simulink model "sraam2023b"  (R2023b)
settings: Solver=ode4  StartTime=0.0  StopTime=25  FixedStep=0.001  RelTol=1e-3
values from neighbouring files (symbols this model uses):
  AEXIT = 0.0125    [SRAAM6_params.m]
  ALIMIT = 50.0    (= 50)    [SRAAM6_params.m]
  ALP_LIMX = 46.0    (= 46)    [SRAAM6_params.m]
  BIASAL = 0.0    (= 0)    [SRAAM6_params.m]
  DDLIMX = 600.0    (= 600)    [SRAAM6_params.m]
  DLIMX = 28.0    (= 28)    [SRAAM6_params.m]
  DPLIMX = 28.0    (= 28)    [SRAAM6_params.m]
  DQLIMX = 28.0    (= 28)    [SRAAM6_params.m]
  DRLIMX = 28.0    (= 28)    [SRAAM6_params.m]
  DT = 0.001    [SRAAM6_params.m]
  EBIASA = zeros(3,1)    [SRAAM6_params.m]
  EBIASG = zeros(3,1)    [SRAAM6_params.m]
  EMISA = zeros(3,1)    [SRAAM6_params.m]
  EMISG = zeros(3,1)    [SRAAM6_params.m]
  ESCALA = zeros(3,1)    [SRAAM6_params.m]
  ESCALG = zeros(3,1)    [SRAAM6_params.m]
  EUNBG = zeros(3,1)    [SRAAM6_params.m]
  FACT_WRCL = 0.0    (= 0)    [SRAAM6_params.m]
  GNAV = 4.0    (= 4)    [SRAAM6_params.m]
  INS_NOISE_PWR_A = 0.0    (= 0)    [SRAAM6_params.m]
  INS_NOISE_PWR_G = 0.0    (= 0)    [SRAAM6_params.m]
  K_ALPHA = 10.0    (= 10)    [SRAAM6_params.m]
  K_BETA = 10.0    (= 10)    [SRAAM6_params.m]
  MINS = 0    [SRAAM6_params.m]
  prop_cg_t = prop_cg_vs_time_t(:)    [SRAAM6_params.m]
  prop_cg_v = prop_cg_vs_time_v(:)    [SRAAM6_params.m]
  prop_mass_t = prop_mass_vs_time_t(:)    [SRAAM6_params.m]
  prop_mass_v = prop_mass_vs_time_v(:)    [SRAAM6_params.m]
  prop_moipitch_t = prop_moipitch_vs_time_t(:)    [SRAAM6_params.m]
  prop_moipitch_v = prop_moipitch_vs_time_v(:)    [SRAAM6_params.m]
  prop_moiroll_t = prop_moiroll_vs_time_t(:)    [SRAAM6_params.m]
  prop_moiroll_v = prop_moiroll_vs_time_v(:)    [SRAAM6_params.m]
  prop_thrust_t = prop_thrust_vs_time_t(:)    [SRAAM6_params.m]
  prop_thrust_v = prop_thrust_vs_time_v(:)    [SRAAM6_params.m]
  REFA = 0.01824    [SRAAM6_params.m]
  REFL = 0.1524    [SRAAM6_params.m]
  SCENARIO = 12    [SRAAM6_params.m]
  TGET_POS_IC = TGET_POS(SCENARIO, :)'    [SRAAM6_params.m]
  TGET_VEL_IC = TGET_VEL(SCENARIO, :)'    [SRAAM6_params.m]
  WBLIMX = 30.0    (= 30)    [SRAAM6_params.m]
  WN_NDI_Q = 50.0    (= 50)    [SRAAM6_params.m]
  WN_NDI_R = 50.0    (= 50)    [SRAAM6_params.m]
  WNACT = 251.0    (= 251)    [SRAAM6_params.m]
  X_IC = [SBEL_INIT; VBEB_IC; Q_IC; OMEGA_IC]    [SRAAM6_params.m]
  XCG_REF = 1.2994    [SRAAM6_params.m]
  ZETACT = 0.7    [SRAAM6_params.m]
  ZRCL = 0.9    [SRAAM6_params.m]
undefined symbols (not defined in the file or in its folder): alpha_bp, beta_bp, ca0_vs_mach, ca0b_vs_mach, caa_vs_mach_alpha_beta, cad_vs_mach, cll0_vs_mach_alpha_beta, clldp_vs_mach_alpha_beta, cllp_vs_mach, clm0_vs_mach_alpha_beta, clmdq_vs_mach_alpha_beta, clmq_vs_mach, cln0_vs_mach_alpha_beta, clndr_vs_mach_alpha_beta, clnr_vs_mach, cn0_vs_mach_alpha_beta, cndq_vs_mach_alpha_beta, cy0_vs_mach_alpha_beta, cydr_vs_mach_alpha_beta, mach_bp
libraries: simulink x3
(part 2 of 2)

== matlab function sraam2023b/Control Subsystem/NDI ==
  data: ancomx input; dqcx output; alcomx input; alphax input; betax input; dvbe input; qqx input; rrx input; fspb2 input; fspb3 input; dna input; dma input; dmq input; dmd input; dyb input; dlnb input; dlnr input; dlnd input; drcx output; ALIMIT parameter; ALP_LIMX parameter; WBLIMX parameter; DQLIMX parameter; DRLIMX parameter; WN_NDI_Q parameter; WN_NDI_R parameter; K_ALPHA parameter; K_BETA parameter
function [dqcx, drcx] = control_ndi( ...
    ancomx, alcomx, ...
    alphax, betax, dvbe, ...
    qqx, rrx, ...
    fspb2, fspb3, ...
    dna, dma, dmq, dmd, dyb, dlnb, dlnr, dlnd, ALIMIT, ALP_LIMX, WBLIMX, DQLIMX, DRLIMX, WN_NDI_Q, WN_NDI_R, K_ALPHA, K_BETA)
% qqx, rrx: deg/s — kinBus'tan direkt
%CONTROL_NDI  Nonlinear Dynamic Inversion — yunuslama + yalpalama.
% Kaynak: missile/control.py — control_ndi()
% Roll ayrı subsystem'de (control_roll.m).
%#codegen

AGRAV  = 9.80665;
DEG    = 180.0 / pi;
RAD    = pi / 180.0;
SMALL  = 1e-7;

alimit   = ALIMIT;
alplimx  = ALP_LIMX;
wblimx   = WBLIMX;
dqlimx   = DQLIMX;
drlimx   = DRLIMX;
wn_ndi_q = WN_NDI_Q;
wn_ndi_r = WN_NDI_R;
k_alpha  = K_ALPHA;
k_beta   = K_BETA;

% ── Yapısal ivme sınırlayıcı ─────────────────────────────────────────────────
aa = sqrt(ancomx^2 + alcomx^2);
if aa > alimit;  aa = alimit;  end
if abs(ancomx) < SMALL && abs(alcomx) < SMALL
    phi_c = 0.0;
else
    phi_c = atan2(ancomx, alcomx);
end
alcomx_l = aa * cos(phi_c);
ancomx_l = aa * sin(phi_c);

% ── ADIM 1: Kuvvet inversiyonu ────────────────────────────────────────────────
dna_s = dna; if abs(dna_s) < SMALL; dna_s = SMALL; end
dyb_s = dyb; if abs(dyb_s) < SMALL; dyb_s = SMALL; end

alpha_cmd = AGRAV * ancomx_l / dna_s;
beta_cmd  = AGRAV * alcomx_l / dyb_s;

alp_lim   = alplimx * RAD;
alpha_cmd = max(min(alpha_cmd, alp_lim), -alp_lim);
beta_cmd  = max(min(beta_cmd,  alp_lim), -alp_lim);

% ── ADIM 2: Kinematik inversiyon ──────────────────────────────────────────────
alpha   = alphax * RAD;
beta    = betax  * RAD;
qq      = qqx * RAD;    % deg/s → rad/s
rr      = rrx * RAD;
V_s     = max(dvbe, 30.0);
an_meas = -fspb3 / AGRAV;
al_meas =  fspb2 / AGRAV;

q_cmd = k_alpha * (alpha_cmd - alpha) + AGRAV * an_meas / V_s;
r_cmd = k_beta  * (beta - beta_cmd)   + AGRAV * al_meas / V_s;

rate_lim = wblimx * RAD;
q_cmd = max(min(q_cmd, rate_lim), -rate_lim);
r_cmd = max(min(r_cmd, rate_lim), -rate_lim);

% ── ADIM 3: Moment inversiyonu ────────────────────────────────────────────────
q_dot_des   = wn_ndi_q * (q_cmd - qq);
r_dot_des   = wn_ndi_r * (r_cmd - rr);
q_dot_model = dma * alpha + dmq * qq;
r_dot_model = dlnb * beta + dlnr * rr;

dmd_s  = dmd;  if abs(dmd_s)  < SMALL; dmd_s  = SMALL; end
dlnd_s = dlnd; if abs(dlnd_s) < SMALL; dlnd_s = SMALL; end

dqc  = (q_dot_des - q_dot_model) / dmd_s;
drc  = (r_dot_des - r_dot_model) / dlnd_s;

dqcx = max(min(dqc * DEG, dqlimx), -dqlimx);
drcx = max(min(drc * DEG, drlimx), -drlimx);
end

== matlab function sraam2023b/Target/Target ==
  data: t input; acc output; pos input; vel input; scenario input
function acc = target_accel(t, pos, vel, scenario)
%TARGET_ACCEL  Hedef ivme vektörü — 10 senaryo.
% Kaynak: missile/target.py — Target._accel()
%
% Girişler:
%   t        : simülasyon zamanı - s
%   pos      : hedef konumu NED - m  (kullanılmıyor, ileriki senaryolar için)
%   vel      : hedef hızı NED - m/s
%   scenario : senaryo numarası (1-10)
%
% Çıkış:
%   acc [3x1]: hedef ivmesi NED - m/s²
%#codegen

G = 9.80665;
acc = zeros(3,1);

vn = vel(1);  ve = vel(2);  vd = vel(3);

% ── Yardımcı: saat yönünde dik vektör (yatay düzlemde) ───────────────────────
vm = sqrt(vn^2 + ve^2);
if vm < 1.0
    cw_n = 0.0;  cw_e = 0.0;
else
    cw_n =  ve / vm;
    cw_e = -vn / vm;
end

if scenario == 1
    % S1: Sabit hız, düz uçuş
    acc = zeros(3,1);

elseif scenario == 2
    % S2: t>1.5s'de 5g sağ kırılma (santripetal)
    if t >= 1.5
        acc = 5.0 * G * [cw_n; cw_e; 0.0];
    end

elseif scenario == 3
    % S3: Sinüsoidal manevra (3g yanal + 2g dikey)
    acc = [0.0; 3.0*G*sin(1.2*t); -2.0*G*cos(1.8*t + pi/3)];

elseif scenario == 4
    % S4: t>2s 8g sağ kırılma, t>3.5s 6g yukarı çekme
    if t >= 4.8
        acc = zeros(3,1);
    elseif t >= 3.5
        acc = [0.0; 0.0; -6.0*G];
    elseif t >= 2.0
        acc = 8.0 * G * [cw_n; cw_e; 0.0];
    end

elseif scenario == 5
    % S5: Sabit hız (beaming)
    acc = zeros(3,1);

elseif scenario == 6
    % S6: t>3s 7g sağ kırılma, t>8s düzleşme
    if t >= 8.0
        acc = zeros(3,1);
    elseif t >= 3.0
        acc = 7.0 * G * [cw_n; cw_e; 0.0];
    end

elseif scenario == 7
    % S7: Sabit hız (look-down)
    acc = zeros(3,1);

elseif scenario == 8
    % S8: t>4s ~9g kombine kırılma
    if t >= 4.0
        acc = [0.0; 6.364*G; -6.364*G];
    end

elseif scenario == 9
    % S9: Afterburner tırmanma (~3g)
    vtot = norm(vel);
    if vtot > 1.0
        vhat = vel / vtot;
        a_drag = -0.7 * G * vhat;
        up = [0.0; 0.0; -1.0];
        perp = up - dot(up, vhat) * vhat;
        pm = norm(perp);
        if pm > 1e-6
            a_lift = 3.0 * G * perp / pm;
        else
            a_lift = zeros(3,1);
        end
        acc = a_drag + a_lift;
    end

elseif scenario == 10
    % S10: 4g koordineli dönüş
    vm2 = sqrt(vn^2 + ve^2);
    if vm2 > 0.1
        ax = -vel(2) / vm2 * 4.0 * G;
        ay =  vel(1) / vm2 * 4.0 * G;
        acc = [ax; ay; 0.0];
    end

elseif scenario == 11
    % S11: 12km + t>7s geç 6g sağ kırılma
    if t >= 7.0
        acc = 6.0 * G * [cw_n; cw_e; 0.0];
    end

elseif scenario == 12
    % S12: 15km + t>5s sinüsoidal jink (3g yanal + 2g dikey)
    if t >= 5.0
        tau = t - 5.0;
        acc = [0.0; 3.0*G*sin(1.0*tau); -2.0*G*cos(1.5*tau)];
    end

elseif scenario == 13
    % S13: Tail-chase + t>4s 7g yukarı + t>6s 7g sağ kırılma
    if t >= 6.0
        acc = 7.0 * G * [cw_n; cw_e; 0.0];
    elseif t >= 4.0
        acc = [0.0; 0.0; -7.0*G];
    end

elseif scenario == 14
    % S14: Uzun beam + t>6s 8g sharp break
    if t >= 6.0
        acc = 8.0 * G * [cw_n; cw_e; 0.0];
    end
end
end

== matlab function sraam2023b/Guidance Subsystem/guidance ==
  data: STEL input; ancomx output; VTEL input; SBELC input; VBELC input; TBL input; alcomx output; dtbc output; tgoc output; GNAV parameter; ALIMIT parameter
function [ancomx, alcomx, dtbc, tgoc] = guidance_pronav( ...
    STEL, VTEL, SBELC, VBELC, TBL, GNAV, ALIMIT)
%GUIDANCE_PRONAV  Orantılı navigasyon güdümü (midcourse pronav).
% Kaynak: missile/guidance.py — _pronav_mid()
%
% Girişler:
%   STEL  [3x1] : hedef konumu NED - m
%   VTEL  [3x1] : hedef hızı NED - m/s
%   SBELC [3x1] : füze konumu (INS tahmini) NED - m
%   VBELC [3x1] : füze hızı (INS tahmini) NED - m/s
%   TBL   [3x3] : gövde-yerel DCM (INS tahmini)
%
% Çıkışlar:
%   ancomx : normal ivme komutu - g
%   alcomx : yanal ivme komutu - g
%   dtbc   : hedefe mesafe - m
%   tgoc   : tahmini uçuş süresi - s
%#codegen

AGRAV = 9.80665;
SMALL = 1e-7;
gnav  = GNAV;     % workspace parametresi
alimit = ALIMIT;  % workspace parametresi

ancomx = 0.0;
alcomx = 0.0;
dtbc   = 0.0;
tgoc   = 0.0;

% ── Hedef-füze görüş vektörü ──────────────────────────────────────────────────
STBLC = STEL - SBELC;
dtbc  = norm(STBLC);

if dtbc < SMALL
    return
end

UTBLC = STBLC / dtbc;

% ── Görüş açısı (diagnostik) ─────────────────────────────────────────────────
% UTBBC = TBL * UTBLC;  (ileride kullanılabilir)

% ── Göreceli hız (hedef - füze) ───────────────────────────────────────────────
VTBLC = VTEL - VBELC;

% ── Kapanma hızı ─────────────────────────────────────────────────────────────
dvtbc = abs(dot(UTBLC, VTBLC));
if dvtbc < SMALL; dvtbc = SMALL; end

% ── Tahmini uçuş süresi ───────────────────────────────────────────────────────
tgoc = dtbc / dvtbc;

% ── Eylemsiz LOS açısal hızı ─────────────────────────────────────────────────
WOELC = cross(UTBLC, VTBLC) / dtbc;

% ── ProNav ivme komutu (gövde ekseni) - g ────────────────────────────────────
ACBX = TBL * cross(WOELC, UTBLC) * gnav * dvtbc / AGRAV;

% ── Yanal ve normal bileşenler ────────────────────────────────────────────────
all_acc =  ACBX(2);
ann_acc = -ACBX(3);

% ── Dairesel sınırlayıcı ─────────────────────────────────────────────────────
aa = sqrt(all_acc^2 + ann_acc^2);
if aa > alimit;  aa = alimit;  end
if abs(ann_acc) < SMALL && abs(all_acc) < SMALL
    phi = 0.0;
else
    phi = atan2(ann_acc, all_acc);
end

alcomx = aa * cos(phi);
ancomx = aa * sin(phi);
end

== matlab function sraam2023b/Hit Condition ==
  data: dtbc input; stop output; t input; HIT_R parameter
function stop = hit_condition(dtbc, t, HIT_R)
%HIT_CONDITION  HIT_R > 0 ise dtbc < HIT_R olduğunda 1 döndürür.
%#codegen

hit_r = HIT_R;   % workspace parametresi (0 = devre dışı)

if hit_r > 0 && dtbc < hit_r && dtbc > 0 && t > 0.1
    stop = 1.0;
else
    stop = 0.0;
end
end

== matlab function sraam2023b/Control Subsystem/NDI-COP ==
  data: ancomx input; dqcx output; alcomx input; alphax input; betax input; dvbe input; qqx input; rrx input; fspb2 input; fspb3 input; dna input; dma input; dmq input; dmd input; dnd input; dyb input; dlnb input; dlnr input; dlnd input; drcx output; ALIMIT parameter; ALP_LIMX parameter; WBLIMX parameter; DQLIMX parameter; DRLIMX parameter; WN_NDI_Q parameter; WN_NDI_R parameter; K_ALPHA parameter; K_BETA parameter
function [dqcx, drcx] = control_ndi_cop( ...
    ancomx, alcomx, ...
    alphax, betax, dvbe, ...
    qqx, rrx, ...
    fspb2, fspb3, ...
    dna, dma, dmq, dmd, dnd, dyb, dlnb, dlnr, dlnd, ALIMIT, ALP_LIMX, WBLIMX, DQLIMX, DRLIMX, WN_NDI_Q, WN_NDI_R, K_ALPHA, K_BETA)
%CONTROL_NDI_COP  NDI autopilot reformulated about the Center of Percussion.
%
% Kaynak: missile/control.py — control_ndi_cop()  (maut=7)
%
% Standart NDI'dan tek fark dış döngüdedir:
%   Standart NDI : alpha_cmd = g*an / dna          (CG referanslı → NMP zero var)
%   NDI-CoP      : alpha_cmd = g*an / dna_cop       (CoP referanslı → NMP zero yok)
%
% CoP konumu (CG'nin önünde, +burun yönü) — m cinsinden:
%   x_cop = -dnd_rad / dmd       dnd_rad = dnd * DEG  [m/s²/deg → m/s²/rad]
%
% CoP'ta efektif kuvvet türevi:
%   dna_cop = dna + x_cop * dma
%   dyb_cop = dyb + x_cop * dlnb
%
% Orta ve iç döngüler standart NDI ile aynıdır.
%
% qqx, rrx: deg/s — kinBus'tan direkt.
%#codegen

AGRAV  = 9.80665;
DEG    = 180.0 / pi;
RAD    = pi / 180.0;
SMALL  = 1e-7;

alimit   = ALIMIT;
alplimx  = ALP_LIMX;
wblimx   = WBLIMX;
dqlimx   = DQLIMX;
drlimx   = DRLIMX;
wn_ndi_q = WN_NDI_Q;
wn_ndi_r = WN_NDI_R;
k_alpha  = K_ALPHA;
k_beta   = K_BETA;

% ── Yapısal ivme sınırlayıcı ─────────────────────────────────────────────────
aa = sqrt(ancomx^2 + alcomx^2);
if aa > alimit;  aa = alimit;  end
if abs(ancomx) < SMALL && abs(alcomx) < SMALL
    phi_c = 0.0;
else
    phi_c = atan2(ancomx, alcomx);
end
alcomx_l = aa * cos(phi_c);
ancomx_l = aa * sin(phi_c);

% ── Center of Percussion ─────────────────────────────────────────────────────
% dnd [m/s²/deg] → [m/s²/rad]: aynı fin açısı için dmd ile birim uyumu sağlanır
dnd_rad = dnd * DEG;

dmd_s  = dmd;  if abs(dmd_s)  < SMALL; dmd_s  = SMALL; end
dlnd_s = dlnd; if abs(dlnd_s) < SMALL; dlnd_s = SMALL; end

% CoP konumu ±3 m ile sınırlandırıldı (düşük q'da sayısal kararlılık)
x_cop_q = max(min(-dnd_rad / dmd_s,  3.0), -3.0);
x_cop_r = max(min(-dnd_rad / dlnd_s, 3.0), -3.0);

% CoP'ta efektif kuvvet türevleri
dna_cop = dna + x_cop_q * dma;
dyb_cop = dyb + x_cop_r * dlnb;

% ── ADIM 1: Kuvvet inversiyonu (CoP referanslı — NMP free) ───────────────────
dna_s = dna_cop; if abs(dna_s) < SMALL; dna_s = SMALL; end
dyb_s = dyb_cop; if abs(dyb_s) < SMALL; dyb_s = SMALL; end

alpha_cmd = AGRAV * ancomx_l / dna_s;
beta_cmd  = AGRAV * alcomx_l / dyb_s;

alp_lim   = alplimx * RAD;
alpha_cmd = max(min(alpha_cmd, alp_lim), -alp_lim);
beta_cmd  = max(min(beta_cmd,  alp_lim), -alp_lim);

% ── ADIM 2: Kinematik inversiyon ──────────────────────────────────────────────
% α̇ = q − (g/V)·aₙ_CG  kimliği CG referanslıdır — an_meas (CG) doğrudur.
alpha   = alphax * RAD;
beta    = betax  * RAD;
qq      = qqx * RAD;    % deg/s → rad/s
rr      = rrx * RAD;
V_s     = max(dvbe, 30.0);
an_meas = -fspb3 / AGRAV;
al_meas =  fspb2 / AGRAV;

q_cmd = k_alpha * (alpha_cmd - alpha) + AGRAV * an_meas / V_s;
r_cmd = k_beta  * (beta - beta_cmd)   + AGRAV * al_meas / V_s;

rate_lim = wblimx * RAD;
q_cmd = max(min(q_cmd, rate_lim), -rate_lim);
r_cmd = max(min(r_cmd, rate_lim), -rate_lim);

% ── ADIM 3: Moment inversiyonu (standart NDI ile aynı) ───────────────────────
q_dot_des   = wn_ndi_q * (q_cmd - qq);
r_dot_des   = wn_ndi_r * (r_cmd - rr);
q_dot_model = dma * alpha + dmq * qq;
r_dot_model = dlnb * beta + dlnr * rr;

dqc  = (q_dot_des - q_dot_model) / dmd_s;
drc  = (r_dot_des - r_dot_model) / dlnd_s;

dqcx = max(min(dqc * DEG, dqlimx), -dqlimx);
drcx = max(min(drc * DEG, drlimx), -drlimx);
end

== matlab function sraam2023b/INS Subsystem/MATLAB Function ==
  data: TBL input; SBELC output; ppx input; qqx input; rrx input; SBEL input; VBEL input; dvbe input; hbe input; fspb1 input; fspb2 input; fspb3 input; RECE input; EVBE input; ESTTC input; noise_g input; noise_a input; noise_h input; VBELC output; TBLC output; ppxc output; qqxc output; rrxc output; fspb2c output; fspb3c output; alphaxc output; betaxc output; dvbec output; hbem output; thtblcx output; phiblcx output; psivlcx output; thtvlcx output; RECED output; EVBED output; ESTTCD output; EBIASG parameter; EBIASA parameter; ESCALG parameter; EMISG parameter; EMISA parameter; EUNBG parameter; BIASAL parameter; ESCALA parameter; MINS parameter
function [SBELC, VBELC, TBLC, ...
          ppxc, qqxc, rrxc, fspb2c, fspb3c, ...
          alphaxc, betaxc, dvbec, hbem, ...
          thtblcx, phiblcx, psivlcx, thtvlcx, ...
          RECED, EVBED, ESTTCD] = ins( ...
    TBL, ppx, qqx, rrx, ...
    SBEL, VBEL, dvbe, hbe, fspb1, fspb2, fspb3, ...
    RECE, EVBE, ESTTC, noise_g, noise_a, noise_h, ...
    EBIASG, EBIASA, ESCALG, EMISG, EMISA, EUNBG, BIASAL, ESCALA, MINS)
%INS  Inertial Navigation System — MINS=0:ideal, MINS=1:gercek IMU.
%   Kaynak: missile/ins.py
%#codegen

DEG   = 180.0 / pi;
RAD   = pi / 180.0;
SMALL = 1e-8;

% ── Tüm çıkışları önceden boyutlandır (Simulink derleme zorunluluğu) ──────────
SBELC   = zeros(3,1);
VBELC   = zeros(3,1);
TBLC    = zeros(3,3);
ppxc    = 0.0;
qqxc    = 0.0;
rrxc    = 0.0;
fspb2c  = 0.0;
fspb3c  = 0.0;
alphaxc = 0.0;
betaxc  = 0.0;
dvbec   = 0.0;
hbem    = 0.0;
thtblcx = 0.0;
phiblcx = 0.0;
psivlcx = 0.0;
thtvlcx = 0.0;
RECED   = zeros(3,1);
EVBED   = zeros(3,1);
ESTTCD  = zeros(3,1);

% ── Gerçek gövde vektörleri ───────────────────────────────────────────────────
WBEB = [ppx; qqx; rrx] * RAD;
FSPB = [fspb1; fspb2; fspb3];

% ── Ideal başlangıç değerleri (MINS=0 için doğrudan kullanılır) ───────────────
SBELC  = [SBEL(1); SBEL(2); SBEL(3)];
VBELC  = [VBEL(1); VBEL(2); VBEL(3)];
TBLC   = TBL;
WBECB  = [WBEB(1); WBEB(2); WBEB(3)];
FSPCB  = [FSPB(1); FSPB(2); FSPB(3)];
dvbec  = dvbe;
hbem   = hbe;

if MINS == 1

    % ── Jiroskop hata modeli ──────────────────────────────────────────────────
    EGB   = diag(ESCALG) + skew3(EMISG);
    EWBEB = EBIASG + EGB * WBEB + EUNBG .* FSPB + noise_g;
    WBECB = WBEB + EWBEB;

    % ── İvmeölçer hata modeli ─────────────────────────────────────────────────
    EAB   = diag(ESCALA) + skew3(EMISA);
    EFSPB = EBIASA + EAB * FSPB;
    FSPCB = FSPB + EFSPB + noise_a;

    % ── Eğim hatası dinamiği: dRECE/dt = TLB * EWBEB ─────────────────────────
    RECED = TBL' * EWBEB;

    % INS DCM: TBLC ≈ TBL * (I + skew(RECE))
    RERE = skew3(RECE);
    TBLC = TBL * (eye(3) + RERE);

    % ── Hız hatası dinamiği ───────────────────────────────────────────────────
    TLCB  = TBLC';
    EVBED = TLCB * EFSPB - RERE * TLCB * FSPCB;

    % ── Konum hatası dinamiği: dESTTC/dt = EVBE ──────────────────────────────
    ESTTCD = EVBE;

    % ── Tahmin birleştirme ────────────────────────────────────────────────────
    SBELC = ESTTC + SBEL;
    VBELC = EVBE  + VBEL;
    dvbec = norm(VBELC);
    hbem  = hbe + BIASAL + noise_h;

end

% ── Türetilmiş tahmin nicelikleri (her iki modda ortak) ───────────────────────
v1 = VBELC(1);  v2 = VBELC(2);  v3 = VBELC(3);
if abs(v1) < SMALL && abs(v2) < SMALL
    psivlc = 0.0;
    thtvlc = 0.0;
else
    psivlc = atan2(v2, v1);
    thtvlc = atan2(-v3, sqrt(v1*v1 + v2*v2));
end

VBEBC  = TBLC * VBELC;
vb1 = VBEBC(1);  vb2 = VBEBC(2);  vb3 = VBEBC(3);
dvbebc = sqrt(vb1*vb1 + vb2*vb2 + vb3*vb3);
if dvbebc < 1e-6;  dvbebc = 1e-6;  end

alphac = atan2(vb3, vb1);
betac  = asin(max(-1.0, min(1.0, vb2 / dvbebc)));

tblc13 = TBLC(1,3);
if abs(tblc13) < 1.0
    thtblc = asin(-tblc13);
elseif tblc13 > 0.0
    thtblc = -pi / 2.0;
else
    thtblc =  pi / 2.0;
end
phiblc = atan2(TBLC(2,3), TBLC(3,3));

% ── Çıkış atamaları ──────────────────────────────────────────────────────────
ppxc    = WBECB(1) * DEG;
qqxc    = WBECB(2) * DEG;
rrxc    = WBECB(3) * DEG;
fspb2c  = FSPCB(2);
fspb3c  = FSPCB(3);
alphaxc = alphac * DEG;
betaxc  = betac  * DEG;
thtblcx = thtblc * DEG;
phiblcx = phiblc * DEG;
psivlcx = psivlc * DEG;
thtvlcx = thtvlc * DEG;

end

function S = skew3(v)
S = [  0.0,  -v(3),  v(2); ...
      v(3),   0.0,  -v(1); ...
     -v(2),   v(1),  0.0 ];
end

== matlab function sraam2023b/kinematics ==
  data: x input; TBL output; alpha_deg output; beta_deg output; alpp_deg output; dvbe output; hbe output; psiblx output; thtblx output; phiblx output; VBEL output; psivlx output; thtvlx output; ppx output; qqx output; rrx output; SBEL output
function [TBL, alpha_deg, beta_deg, alpp_deg, dvbe, hbe, ...
          psiblx, thtblx, phiblx, VBEL, psivlx, thtvlx, ...
          ppx, qqx, rrx, SBEL] = ...
          state_to_outputs(x)
%STATE_TO_OUTPUTS  x[13] vektöründen ikincil çıkışları hesaplar.
% Algebraic — integratör yok. Simulink MATLAB Function bloğuna koy.
%
% Kaynak: kinematics.py:144-235, newton.py:107-157
%#codegen

EPS   = 1e-10;
DEG   = 180.0 / pi;
SMALL = 1e-7;

% Durumu aç
SBEL = x(1:3);
VBEB = x(4:6);
q    = x(7:10);
om   = x(11:13);

q0=q(1); q1=q(2); q2=q(3); q3=q(4);

% ── DCM ──────────────────────────────────────────────────────────────────────
TBL = [ q0^2+q1^2-q2^2-q3^2,  2*(q1*q2+q0*q3),  2*(q1*q3-q0*q2);
        2*(q1*q2-q0*q3),  q0^2-q1^2+q2^2-q3^2,  2*(q2*q3+q0*q1);
        2*(q1*q3+q0*q2),  2*(q2*q3-q0*q1),  q0^2-q1^2-q2^2+q3^2];

% ── Euler Açıları (kinematics.py:159-185) ────────────────────────────────────
tbl13 = TBL(1,3);
if abs(tbl13) < 1.0
    thtbl = asin(-tbl13);
else
    thtbl = pi/2 * sign(-tbl13);
end
cthtbl = max(cos(thtbl), EPS);

cpsi = TBL(1,1) / cthtbl;
cpsi = max(min(cpsi, 1-EPS), -(1-EPS));
cphi = TBL(3,3) / cthtbl;
cphi = max(min(cphi, 1-EPS), -(1-EPS));

psibl = acos(cpsi) * sign(TBL(1,2));
phibl = acos(cphi) * sign(TBL(2,3));

psiblx = psibl * DEG;
thtblx = thtbl * DEG;
phiblx = phibl * DEG;

% ── NED Hızı ve Hız ──────────────────────────────────────────────────────────
VBEL = TBL' * VBEB;
vbel1 = VBEL(1);  vbel2 = VBEL(2);  vbel3 = VBEL(3);
dvbe  = norm(VBEL);
if dvbe < EPS; dvbe = EPS; end

% ── Uçuş yolu açıları ────────────────────────────────────────────────────────
if abs(vbel1) < SMALL && abs(vbel2) < SMALL
    psivlx = 0.0;
else
    psivlx = atan2(vbel2, vbel1) * DEG;
end
thtvlx = atan2(-vbel3, sqrt(vbel1^2 + vbel2^2)) * DEG;

% ── İrtifa ────────────────────────────────────────────────────────────────────
hbe = -SBEL(3);

% ── Hücum ve kayma açıları (kinematics.py:187-215) ───────────────────────────
vbeb1 = VBEB(1);  vbeb2 = VBEB(2);  vbeb3 = VBEB(3);

alpha_rad = atan2(vbeb3, vbeb1);
beta_rad  = asin(max(-1.0, min(1.0, vbeb2 / dvbe)));

dum = vbeb1 / dvbe;
dum = max(min(dum, 1-EPS), -(1-EPS));
alpp_rad = acos(dum);

alpha_deg = alpha_rad * DEG;
beta_deg  = beta_rad  * DEG;
alpp_deg  = alpp_rad  * DEG;

% ── Açısal hızlar (x(11:13) rad/s → deg/s) ───────────────────────────────────
ppx = x(11) * DEG;
qqx = x(12) * DEG;
rrx = x(13) * DEG;

% ── Konum (Guidance için) ─────────────────────────────────────────────────────
SBEL = x(1:3);
end

== matlab function sraam2023b/6-DOF ==
  data: x input; xdot output; FAPB input; FMB input; grav input; mass input; ai11 input; ai33 input
function xdot = six_dof_deriv(x, FAPB, FMB, grav, mass, ai11, ai33)
%
% Girişler:
%   x     [13x1]  Durum vektörü: [SBEL(3); VBEB(3); q(4); omega(3)]
%   FAPB  [3x1]   Yerçekimi dışı toplam kuvvet, gövde ekseni - N
%   FMB   [3x1]   Toplam moment, gövde ekseni - N·m
%   mass  [1]     Araç kütlesi - kg
%   grav  [1]     Yerçekimi ivmesi - m/s²
%   ai11  [1]     Yuvarlanma atalet momenti - kg·m²
%   ai33  [1]     Yunuslama/yalpalama atalet momenti - kg·m²
%
% Çıkışlar:
%   xdot  [13x1]  Durum türevi: dx/dt
%#codegen

% ── Durumu aç ────────────────────────────────────────────────────────────────
SBEL = x(1:3);   % konum NED - m         (kullanılmıyor, sadece türevi var)
VBEB = x(4:6);   % hız gövde ekseni - m/s
q    = x(7:10);  % quaternion [q0;q1;q2;q3]
om   = x(11:13); % açısal hız [p;q;r] - rad/s
xdot = zeros(13, 1);
pp = om(1);  qq_r = om(2);  rr = om(3);

% ── Quaternion → DCM (kinematics.py:145-149) ─────────────────────────────────
q0 = q(1);  q1 = q(2);  q2 = q(3);  q3 = q(4);
TBL = [ q0^2+q1^2-q2^2-q3^2,  2*(q1*q2+q0*q3),  2*(q1*q3-q0*q2);
        2*(q1*q2-q0*q3),  q0^2-q1^2+q2^2-q3^2,  2*(q2*q3+q0*q1);
        2*(q1*q3+q0*q2),  2*(q2*q3-q0*q1),  q0^2-q1^2-q2^2+q3^2];

% ── Konum türevi: dSBEL/dt = TBL' * VBEB (newton.py:101) ────────────────────
dSBEL = TBL' * VBEB;

% ── Hız türevi: Newton 2. kanun dönen çerçevede (newton.py:84-94) ────────────
FSPB  = FAPB / mass;                       % spesifik kuvvet - m/s²
ATB   = cross(om, VBEB);                   % Coriolis: ω × V
dVBEB = FSPB - ATB + TBL * [0; 0; grav];  % grav NED aşağı pozitif

% ── Quaternion türevi (kinematics.py:127-135) ─────────────────────────────────
ck = 50.0;                                 % ortogonalite düzeltme kazancı
ortho_err = 1.0 - dot(q, q);
Omega = [  0,   -pp, -qq_r, -rr;
           pp,   0,   rr,  -qq_r;
           qq_r, -rr,  0,    pp;
           rr,   qq_r, -pp,   0 ];
dq = 0.5 * Omega * q + ck * ortho_err * q;

% ── Açısal hız türevi: Euler denklemleri (euler.py:45-47) ────────────────────
dpp = FMB(1) / ai11;
dqq = ((ai33 - ai11) * pp * rr + FMB(2)) / ai33;
drr = (-(ai33 - ai11) * pp * qq_r + FMB(3)) / ai33;

% ── Paketle ───────────────────────────────────────────────────────────────────
xdot = [dSBEL; dVBEB; dq; dpp; dqq; drr];
end
